simulink model "milestone2"  (R2013b)
settings: Solver=ode45  StartTime=0.0  StopTime=10.0  RelTol=1e-3
settings Model: Creator=YinyiChen  LastModifiedBy=YinyiChen

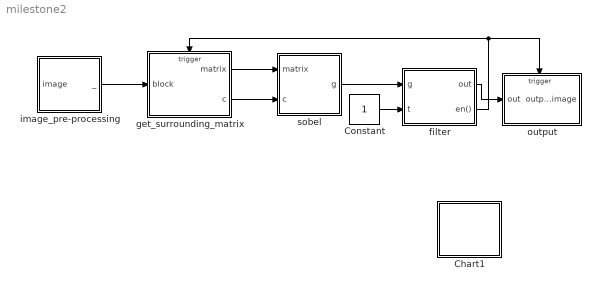
== system milestone2 ==
  Chart1 : Stateflow chart  TreatAsAtomicUnit=on
  Constant : Constant
  filter : Stateflow chart  TreatAsAtomicUnit=on
  get_surrounding_matrix : Stateflow chart  TreatAsAtomicUnit=on
  image_pre-processing : Stateflow chart  TreatAsAtomicUnit=on
  output : Stateflow chart  TreatAsAtomicUnit=on
  "sobel " : Stateflow chart  TreatAsAtomicUnit=on
  wires:
  image_pre-processing/1(_) -> get_surrounding_matrix/1(block)
  get_surrounding_matrix/1(matrix) -> "sobel "/1(matrix)
  "sobel "/1(g) -> filter/1(g)
  Constant/1 -> filter/2(t)
  get_surrounding_matrix/2(c) -> "sobel "/2(c)
  filter/2(en()) -> get_surrounding_matrix/Trigger, output/Trigger
  filter/1(out) -> output/1(out)

== stateflow chart milestone2/image_pre-processing ==
  data: image input; _ output double

== stateflow chart milestone2/get_surrounding_matrix ==
  data: block input; matrix output double; c output double
  events: en input RISING_EDGE_EVENT

== stateflow chart milestone2/sobel  ==
  data: matrix input; g output double; c input

== stateflow chart milestone2/filter ==
  data: g input; t input; out output double
  events: en output FUNCTION_CALL_EVENT

== stateflow chart milestone2/output ==
  data: out input; output_image output double
  events: finish input RISING_EDGE_EVENT

== stateflow chart milestone2/Chart1 ==
